simulink model "diosya"  (R2022a)
settings: Solver=FixedStepAuto  StartTime=0.0  StopTime=10.0  RelTol=1e-3
libraries: vexv5lib x61, vexcommonlib x1
settings Model: Creator=alice  LastModifiedBy=alice
settings SolverCC: AlgebraicLoopSolver=TrustRegion
settings DataIOCC: ReturnWorkspaceOutputs=off
settings OptimizationCC: EnhancedBackFolding=on  PassReuseOutputArgsAs=Individual arguments  MaxStackSize=64  OptimizeBlockOrder=speed  DifferentSizesBufferReuse=on  OptimizationCustomize=off  EfficientTunableParamExpr=on
settings DebuggingCC: ParameterTunabilityLossMsg=error  UnconnectedInputMsg=warning  UnconnectedOutputMsg=warning  UnconnectedLineMsg=warning  SFMachineParentedDataDiag=warning  ArithmeticOperatorsInVariantConditions=warning
settings HardwareCC: ProdBitPerPointer=32  ProdBitPerSizeT=32  ProdBitPerPtrDiffT=32  ProdLargestAtomicInteger=Long  ProdLargestAtomicFloat=Double  ProdWordSize=32  ProdHWDeviceType=ARM Compatible->ARM Cortex
settings SFSimCC: MATLABDynamicMemAlloc=off  CustomCodeUndefinedFunction=UseInterfaceOnly
settings RTWCC: SystemTargetFile=ert.tlc  HardwareBoard=VEX V5 Robot Brain  TLCOptions="-aInlineSetEventsForThisBaseRateFcn=TLC_FALSE -aSuppressMultiTaskScheduler=TLC_FALSE  -aRateBasedStepFcn=0"  TemplateMakefile=ert_default_tmf  GenerateReport=on  Toolchain=GNU Tools for ARM Embedded Processors  IncludeHyperlinkInReport=on  LaunchReport=on  GenerateTraceInfo=on  GenerateTraceReport=on  GenerateTraceReportSl=on  GenerateTraceReportSf=on  GenerateTraceReportEml=on
settings CodeAppCC: ForceParamTrailComments=on  IgnoreCustomStorageClasses=off  OperatorAnnotations=on  SimulinkDataObjDesc=on  SFDataObjDesc=on  InsertBlockDesc=on

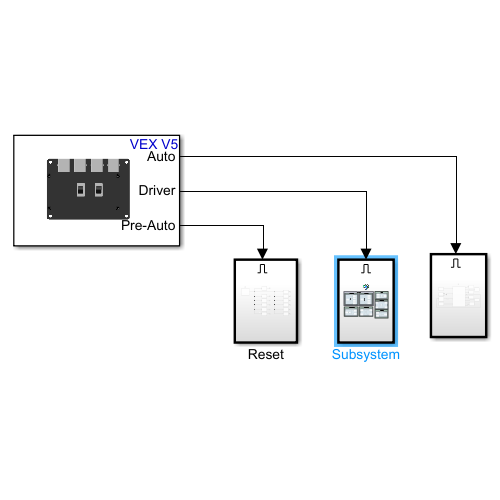
[thumbnail: Simulink's stored preview of the top-level diagram]
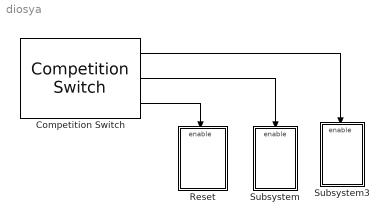
== system diosya ==
  Competition Switch : vexv5lib/Gamepad/Competition Switch  SampleTime=0.02
      settings: SourceProductBaseCode=VEXV5
  Reset : Subsystem
  Subsystem : Subsystem
  Subsystem3 : Subsystem
  wires:
  Competition Switch/1 -> Subsystem3/Enable
  Competition Switch/2 -> Subsystem/Enable
  Competition Switch/3 -> Reset/Enable

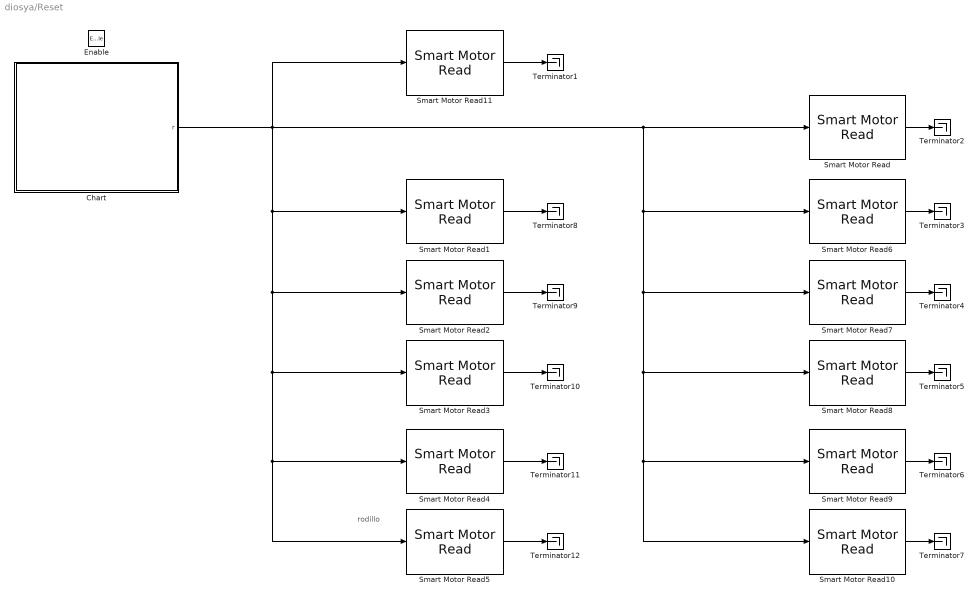
== system diosya/Reset ==
  note: rodillo
  Enable : EnablePort
  Chart : Stateflow chart  TreatAsAtomicUnit=on
  Smart Motor Read : vexv5lib/Sensors/Smart Motor Read  motorPort=2  EncoderUnit=Counts  resetOption=Reset by external signal  additionalOutput=off  SampleTime=0.2
      settings: SourceProductBaseCode=VEXV5
  Smart Motor Read1 : vexv5lib/Sensors/Smart Motor Read  motorPort=10  EncoderUnit=Degrees  resetOption=Reset by external signal  additionalOutput=off  SampleTime=0.2
      settings: SourceProductBaseCode=VEXV5
  Smart Motor Read10 : vexv5lib/Sensors/Smart Motor Read  motorPort=14  EncoderUnit=Degrees  resetOption=Reset by external signal  additionalOutput=off  SampleTime=0.2
      settings: SourceProductBaseCode=VEXV5
  Smart Motor Read11 : vexv5lib/Sensors/Smart Motor Read  motorPort=18  EncoderUnit=Counts  resetOption=Reset by external signal  additionalOutput=off  SampleTime=0.2
      settings: SourceProductBaseCode=VEXV5
  Smart Motor Read2 : vexv5lib/Sensors/Smart Motor Read  motorPort=8  EncoderUnit=Degrees  resetOption=Reset by external signal  additionalOutput=off  SampleTime=0.2
      settings: SourceProductBaseCode=VEXV5
  Smart Motor Read3 : vexv5lib/Sensors/Smart Motor Read  motorPort=9  EncoderUnit=Degrees  resetOption=Reset by external signal  additionalOutput=off  SampleTime=0.2
      settings: SourceProductBaseCode=VEXV5
  Smart Motor Read4 : vexv5lib/Sensors/Smart Motor Read  motorPort=19  EncoderUnit=Degrees  resetOption=Reset by external signal  additionalOutput=off  SampleTime=0.2
      settings: SourceProductBaseCode=VEXV5
  Smart Motor Read5 : vexv5lib/Sensors/Smart Motor Read  motorPort=3  EncoderUnit=Degrees  resetOption=Reset by external signal  additionalOutput=off  SampleTime=0.2
      settings: SourceProductBaseCode=VEXV5
  Smart Motor Read6 : vexv5lib/Sensors/Smart Motor Read  motorPort=7  EncoderUnit=Degrees  resetOption=Reset by external signal  additionalOutput=off  SampleTime=0.2
      settings: SourceProductBaseCode=VEXV5
  Smart Motor Read7 : vexv5lib/Sensors/Smart Motor Read  motorPort=12  EncoderUnit=Degrees  resetOption=Reset by external signal  additionalOutput=off  SampleTime=0.2
      settings: SourceProductBaseCode=VEXV5
  Smart Motor Read8 : vexv5lib/Sensors/Smart Motor Read  motorPort=13  EncoderUnit=Degrees  resetOption=Reset by external signal  additionalOutput=off  SampleTime=0.2
      settings: SourceProductBaseCode=VEXV5
  Smart Motor Read9 : vexv5lib/Sensors/Smart Motor Read  motorPort=17  EncoderUnit=Degrees  resetOption=Reset by external signal  additionalOutput=off  SampleTime=0.2
      settings: SourceProductBaseCode=VEXV5
  Terminator{1..12} (12 alike) : Terminator
  wires:
  Smart Motor Read/1 -> Terminator2/1
  Chart/1(r) -> Smart Motor Read5/1, Smart Motor Read4/1, Smart Motor Read3/1, Smart Motor Read2/1, Smart Motor Read1/1, Smart Motor Read11/1, Smart Motor Read6/1, Smart Motor Read9/1, Smart Motor Read10/1, Smart Motor Read8/1, Smart Motor Read7/1, Smart Motor Read/1
  Smart Motor Read8/1 -> Terminator5/1
  Smart Motor Read4/1 -> Terminator11/1
  Smart Motor Read1/1 -> Terminator8/1
  Smart Motor Read3/1 -> Terminator10/1
  Smart Motor Read9/1 -> Terminator6/1
  Smart Motor Read2/1 -> Terminator9/1
  Smart Motor Read5/1 -> Terminator12/1
  Smart Motor Read10/1 -> Terminator7/1
  Smart Motor Read7/1 -> Terminator4/1
  Smart Motor Read6/1 -> Terminator3/1
  Smart Motor Read11/1 -> Terminator1/1

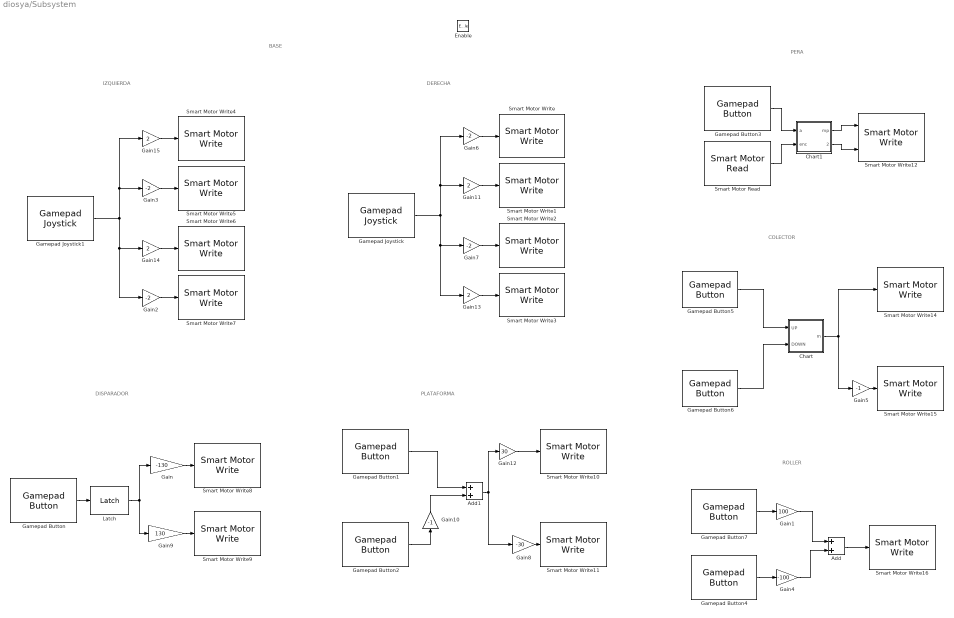
== system diosya/Subsystem ==
  note: PERA
  note: DISPARADOR
  note: DERECHA
  note: ROLLER
  note: BASE
  note: PLATAFORMA
  note: IZQUIERDA
  note: COLECTOR
  Enable : EnablePort
  Add : Sum
  Add1 : Sum
  Chart : Stateflow chart  TreatAsAtomicUnit=on
      settings: PortSchema="{\"entries\":[{\"content\":{\"sides\":[{\"content\":{\"connectorIds\":[\"In2\",\"In1\"]},\"type\":\"ConnectorPlacement.EquallySpacedRectSide\",\"uuid\":\"cbee530c-459d-43ce-b0ca-bbbcd9764774\"},{\"content\":{\"connectorIds\":[\"Out1\"],\"side\":\"RIGHT\"},\"type\":\"ConnectorPlacement.EquallySpacedRectSide\",\"uuid\":\"d644d29c-22a6-445b-a79a-ab4f9a428935\"},{\"content\":{\"connectorIds\":[],\"side\":\"TOP\"},\"type\":\"ConnectorPlacement.EquallySpacedRectSide\",\"uuid\":\"bec18bfc-fa48-4772-9326-1d1444bb53f6\"}]},\"type\":\"ConnectorPlacement.EquallySpacedConnector\",\"uuid\":\"71acd1fe-ef1f-429a-bb10-23fe236c7399\"}],\"packageUris\":[\"http://schema.mathworks.com/mf0/Connector/R2020b\"],\"version\":\"1.0\"}"
  Chart1 : Stateflow chart  TreatAsAtomicUnit=on
  Gain : Gain  Gain=-130
  Gain1 : Gain  Gain=100
  Gain10 : Gain  Gain=-1
  Gain{11,13..15} (4 alike) : Gain  Gain=2
  Gain12 : Gain  Gain=30
  Gain{2..3,6..7} (4 alike) : Gain  Gain=-2
  Gain4 : Gain  Gain=-100
  Gain5 : Gain  Gain=-1
  Gain8 : Gain  Gain=-30
  Gain9 : Gain  Gain=130
  Gamepad Button : vexv5lib/Gamepad/Gamepad Button  joystickType=Primary  chan=A  SampleTime=0.02
      settings: SourceProductBaseCode=VEXV5
  Gamepad Button1 : vexv5lib/Gamepad/Gamepad Button  joystickType=Primary  chan=L1  SampleTime=0.02
      settings: SourceProductBaseCode=VEXV5
  Gamepad Button2 : vexv5lib/Gamepad/Gamepad Button  joystickType=Primary  chan=R1  SampleTime=0.02
      settings: SourceProductBaseCode=VEXV5
  Gamepad Button3 : vexv5lib/Gamepad/Gamepad Button  joystickType=Primary  chan=X  SampleTime=0.02
      settings: SourceProductBaseCode=VEXV5
  Gamepad Button4 : vexv5lib/Gamepad/Gamepad Button  joystickType=Primary  chan=R2  SampleTime=0.02
      settings: SourceProductBaseCode=VEXV5
  Gamepad Button5 : vexv5lib/Gamepad/Gamepad Button  joystickType=Primary  chan=B  SampleTime=0.02
      settings: SourceProductBaseCode=VEXV5
  Gamepad Button6 : vexv5lib/Gamepad/Gamepad Button  joystickType=Primary  chan=DOWN  SampleTime=0.02
      settings: SourceProductBaseCode=VEXV5
  Gamepad Button7 : vexv5lib/Gamepad/Gamepad Button  joystickType=Primary  chan=L2  SampleTime=0.02
      settings: SourceProductBaseCode=VEXV5
  Gamepad Joystick : vexv5lib/Gamepad/Gamepad Joystick  joystickType=Primary  chan=2  SampleTime=0.02
      settings: SourceProductBaseCode=VEXV5
  Gamepad Joystick1 : vexv5lib/Gamepad/Gamepad Joystick  joystickType=Primary  chan=3  SampleTime=0.02
      settings: SourceProductBaseCode=VEXV5
  Latch : vexcommonlib/Latch  output0=off  BlockPlatform=vexv5
      settings: SourceProductBaseCode=EC_VEX_MICRO,VEXV5
  Smart Motor Read : vexv5lib/Sensors/Smart Motor Read  motorPort=18  EncoderUnit=Counts  resetOption=No reset  additionalOutput=off  SampleTime=0.2
      settings: SourceProductBaseCode=VEXV5
  Smart Motor Write : vexv5lib/Actuators/Smart Motor Write  motorPort=2  scaleFactor=18:1  MotorBrakeMode=Coast  OperationMode=Velocity Control
      settings: SourceProductBaseCode=VEXV5
  Smart Motor Write1 : vexv5lib/Actuators/Smart Motor Write  motorPort=7  scaleFactor=18:1  MotorBrakeMode=Coast  OperationMode=Velocity Control
      settings: SourceProductBaseCode=VEXV5
  Smart Motor Write10 : vexv5lib/Actuators/Smart Motor Write  motorPort=17  scaleFactor=36:1  MotorBrakeMode=Hold  OperationMode=Velocity Control
      settings: SourceProductBaseCode=VEXV5
  Smart Motor Write11 : vexv5lib/Actuators/Smart Motor Write  motorPort=14  scaleFactor=36:1  MotorBrakeMode=Hold  OperationMode=Velocity Control
      settings: SourceProductBaseCode=VEXV5
  Smart Motor Write12 : vexv5lib/Actuators/Smart Motor Write  motorPort=18  scaleFactor=18:1  MotorBrakeMode=Coast  OperationMode=Position Control
      settings: SourceProductBaseCode=VEXV5
  Smart Motor Write14 : vexv5lib/Actuators/Smart Motor Write  motorPort=16  scaleFactor=18:1  MotorBrakeMode=Coast  OperationMode=Velocity Control
      settings: SourceProductBaseCode=VEXV5
  Smart Motor Write15 : vexv5lib/Actuators/Smart Motor Write  motorPort=11  scaleFactor=18:1  MotorBrakeMode=Coast  OperationMode=Velocity Control
      settings: SourceProductBaseCode=VEXV5
  Smart Motor Write16 : vexv5lib/Actuators/Smart Motor Write  motorPort=3  scaleFactor=18:1  MotorBrakeMode=Coast  OperationMode=Velocity Control
      settings: SourceProductBaseCode=VEXV5
  Smart Motor Write2 : vexv5lib/Actuators/Smart Motor Write  motorPort=12  scaleFactor=18:1  MotorBrakeMode=Coast  OperationMode=Velocity Control
      settings: SourceProductBaseCode=VEXV5
  Smart Motor Write3 : vexv5lib/Actuators/Smart Motor Write  motorPort=13  scaleFactor=18:1  MotorBrakeMode=Coast  OperationMode=Velocity Control
      settings: SourceProductBaseCode=VEXV5
  Smart Motor Write4 : vexv5lib/Actuators/Smart Motor Write  motorPort=10  scaleFactor=18:1  MotorBrakeMode=Coast  OperationMode=Velocity Control
      settings: SourceProductBaseCode=VEXV5
  Smart Motor Write5 : vexv5lib/Actuators/Smart Motor Write  motorPort=8  scaleFactor=18:1  MotorBrakeMode=Coast  OperationMode=Velocity Control
      settings: SourceProductBaseCode=VEXV5
  Smart Motor Write6 : vexv5lib/Actuators/Smart Motor Write  motorPort=9  scaleFactor=18:1  MotorBrakeMode=Coast  OperationMode=Velocity Control
      settings: SourceProductBaseCode=VEXV5
  Smart Motor Write7 : vexv5lib/Actuators/Smart Motor Write  motorPort=19  scaleFactor=18:1  MotorBrakeMode=Coast  OperationMode=Velocity Control
      settings: SourceProductBaseCode=VEXV5
  Smart Motor Write8 : vexv5lib/Actuators/Smart Motor Write  motorPort=20  scaleFactor=18:1  MotorBrakeMode=Coast  OperationMode=Velocity Control
      settings: SourceProductBaseCode=VEXV5
  Smart Motor Write9 : vexv5lib/Actuators/Smart Motor Write  motorPort=4  scaleFactor=18:1  MotorBrakeMode=Coast  OperationMode=Velocity Control
      settings: SourceProductBaseCode=VEXV5
  wires:
  Gamepad Joystick1/1 -> Gain14/1, Gain2/1, Gain3/1, Gain15/1
  Gain9/1 -> Smart Motor Write9/1
  Gamepad Button4/1 -> Gain4/1
  Add1/1 -> Gain8/1, Gain12/1
  Gamepad Button/1 -> Latch/1
  Gain1/1 -> Add/1
  Gain4/1 -> Add/2
  Chart/1(m) -> Gain5/1, Smart Motor Write14/1
  Add/1 -> Smart Motor Write16/1
  Gamepad Button7/1 -> Gain1/1
  Gain10/1 -> Add1/2
  Gain14/1 -> Smart Motor Write6/1
  Gamepad Button6/1 -> Chart/1(DOWN)
  Gain7/1 -> Smart Motor Write2/1
  Gain11/1 -> Smart Motor Write1/1
  Gain13/1 -> Smart Motor Write3/1
  Gamepad Joystick/1 -> Gain7/1, Gain13/1, Gain11/1, Gain6/1
  Gain8/1 -> Smart Motor Write11/1
  Gamepad Button2/1 -> Gain10/1
  Gain/1 -> Smart Motor Write8/1
  Gain3/1 -> Smart Motor Write5/1
  Gamepad Button3/1 -> Chart1/1(a)
  Gain5/1 -> Smart Motor Write15/1
  Latch/1 -> Gain9/1, Gain/1
  Gamepad Button5/1 -> Chart/2(UP)
  Chart1/1(mp) -> Smart Motor Write12/1
  Chart1/2(position) -> Smart Motor Write12/2
  Smart Motor Read/1 -> Chart1/2(enc)
  Gain15/1 -> Smart Motor Write4/1
  Gain12/1 -> Smart Motor Write10/1
  Gamepad Button1/1 -> Add1/1
  Gain2/1 -> Smart Motor Write7/1
  Gain6/1 -> Smart Motor Write/1

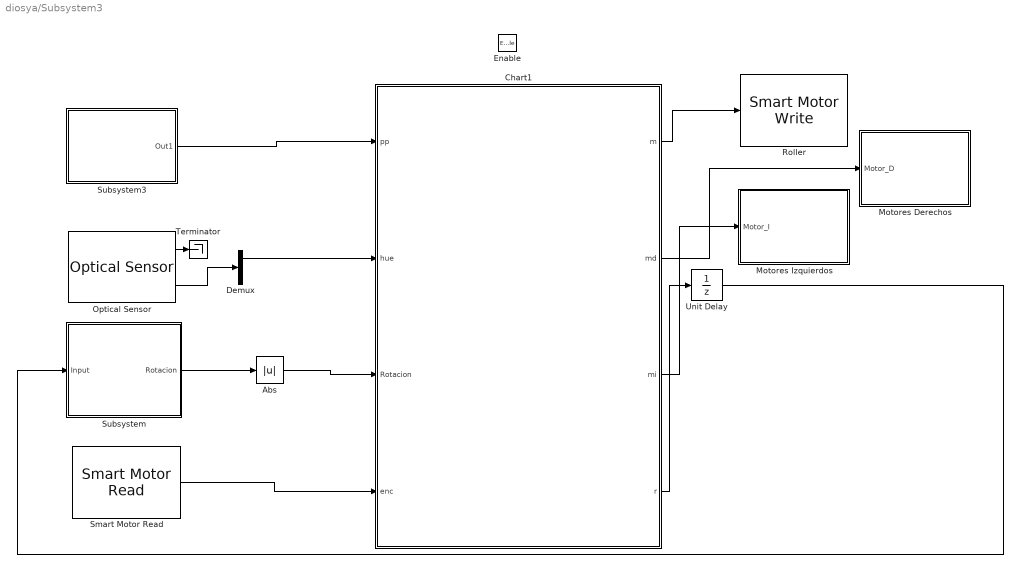
== system diosya/Subsystem3 ==
  Enable : EnablePort
  Abs : Abs  SaturateOnIntegerOverflow=off
  Chart1 : Stateflow chart  TreatAsAtomicUnit=on
      settings: PortSchema="{\"entries\":[{\"content\":{\"sides\":[{\"content\":{\"connectorIds\":[\"In4\",\"In1\",\"In2\",\"In3\"]},\"type\":\"ConnectorPlacement.EquallySpacedRectSide\",\"uuid\":\"6dcbe489-9116-465f-8670-0b6fb9f421dc\"},{\"content\":{\"connectorIds\":[\"Out1\",\"Out2\",\"Out3\",\"Out4\"],\"side\":\"RIGHT\"},\"type\":\"ConnectorPlacement.EquallySpacedRectSide\",\"uuid\":\"705a66a0-558e-4373-baaf-984c25ba8fc1\"},{\"content\":{\"connectorIds\":[],\"side\":\"TOP\"},\"type\":\"ConnectorPlacement.EquallySpacedRectSide\",\"uuid\":\"a9acb6ac-8695-4fbf-8ec3-a93009f982d4\"}]},\"type\":\"ConnectorPlacement.EquallySpacedConnector\",\"uuid\":\"5cef7c66-f869-485c-ad0a-97aa792678b1\"}],\"packageUris\":[\"http://schema.mathworks.com/mf0/Connector/R2020b\"],\"version\":\"1.0\"}"
  Demux : Demux  Outputs=3
  Motores Derechos : Subsystem
  Motores Izquierdos : Subsystem
  Optical Sensor : vexv5lib/Sensors/Optical Sensor  SmartPort=15  Mode=Color  LedPower=100.0  HSBopt=on  RGBopt=off  RawGestureOpt=off  SampleTime=0.1
      settings: SourceProductBaseCode=VEXV5
  Roller : vexv5lib/Actuators/Smart Motor Write  motorPort=3  scaleFactor=18:1  MotorBrakeMode=Brake  OperationMode=Velocity Control
      settings: SourceProductBaseCode=VEXV5
  Smart Motor Read : vexv5lib/Sensors/Smart Motor Read  motorPort=18  EncoderUnit=Counts  resetOption=No reset  additionalOutput=off  SampleTime=0.2
      settings: SourceProductBaseCode=VEXV5
  Subsystem : Subsystem
  Subsystem3 : Subsystem
  Terminator : Terminator
  Unit Delay : UnitDelay  SampleTime=-1  HasFrameUpgradeWarning=on
  wires:
  Chart1/1(m) -> Roller/1
  Optical Sensor/2 -> Demux/1
  Demux/1 -> Chart1/1(hue)
  Optical Sensor/1 -> Terminator/1
  Chart1/2(md) -> Motores Derechos/1(Motor_D)
  Chart1/3(mi) -> Motores Izquierdos/1(Motor_I)
  Subsystem/1(Rotacion) -> Abs/1
  Abs/1 -> Chart1/2(Rotacion)
  Chart1/4(r) -> Unit Delay/1
  Unit Delay/1 -> Subsystem/1(Input)
  Smart Motor Read/1 -> Chart1/3(enc)
  Subsystem3/1(Out1) -> Chart1/4(pp)

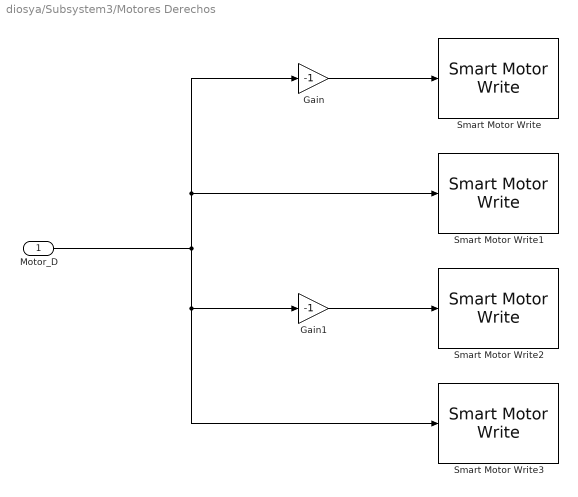
== system diosya/Subsystem3/Motores Derechos ==
  Motor_D : Inport
  Gain : Gain  Gain=-1
  Gain1 : Gain  Gain=-1
  Smart Motor Write : vexv5lib/Actuators/Smart Motor Write  motorPort=2  scaleFactor=36:1  MotorBrakeMode=Brake  OperationMode=Velocity Control
      settings: SourceProductBaseCode=VEXV5
  Smart Motor Write1 : vexv5lib/Actuators/Smart Motor Write  motorPort=7  scaleFactor=36:1  MotorBrakeMode=Brake  OperationMode=Velocity Control
      settings: SourceProductBaseCode=VEXV5
  Smart Motor Write2 : vexv5lib/Actuators/Smart Motor Write  motorPort=12  scaleFactor=36:1  MotorBrakeMode=Brake  OperationMode=Velocity Control
      settings: SourceProductBaseCode=VEXV5
  Smart Motor Write3 : vexv5lib/Actuators/Smart Motor Write  motorPort=13  scaleFactor=36:1  MotorBrakeMode=Brake  OperationMode=Velocity Control
      settings: SourceProductBaseCode=VEXV5
  wires:
  Motor_D/1 -> Smart Motor Write3/1, Gain1/1, Smart Motor Write1/1, Gain/1
  Gain/1 -> Smart Motor Write/1
  Gain1/1 -> Smart Motor Write2/1

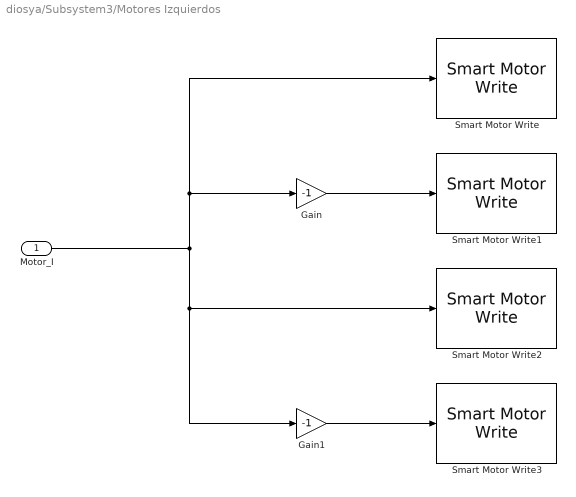
== system diosya/Subsystem3/Motores Izquierdos ==
  Motor_I : Inport
  Gain : Gain  Gain=-1
  Gain1 : Gain  Gain=-1
  Smart Motor Write : vexv5lib/Actuators/Smart Motor Write  motorPort=10  scaleFactor=36:1  MotorBrakeMode=Brake  OperationMode=Velocity Control
      settings: SourceProductBaseCode=VEXV5
  Smart Motor Write1 : vexv5lib/Actuators/Smart Motor Write  motorPort=8  scaleFactor=36:1  MotorBrakeMode=Brake  OperationMode=Velocity Control
      settings: SourceProductBaseCode=VEXV5
  Smart Motor Write2 : vexv5lib/Actuators/Smart Motor Write  motorPort=9  scaleFactor=36:1  MotorBrakeMode=Brake  OperationMode=Velocity Control
      settings: SourceProductBaseCode=VEXV5
  Smart Motor Write3 : vexv5lib/Actuators/Smart Motor Write  motorPort=19  scaleFactor=36:1  MotorBrakeMode=Brake  OperationMode=Velocity Control
      settings: SourceProductBaseCode=VEXV5
  wires:
  Motor_I/1 -> Gain1/1, Smart Motor Write2/1, Gain/1, Smart Motor Write/1
  Gain/1 -> Smart Motor Write1/1
  Gain1/1 -> Smart Motor Write3/1

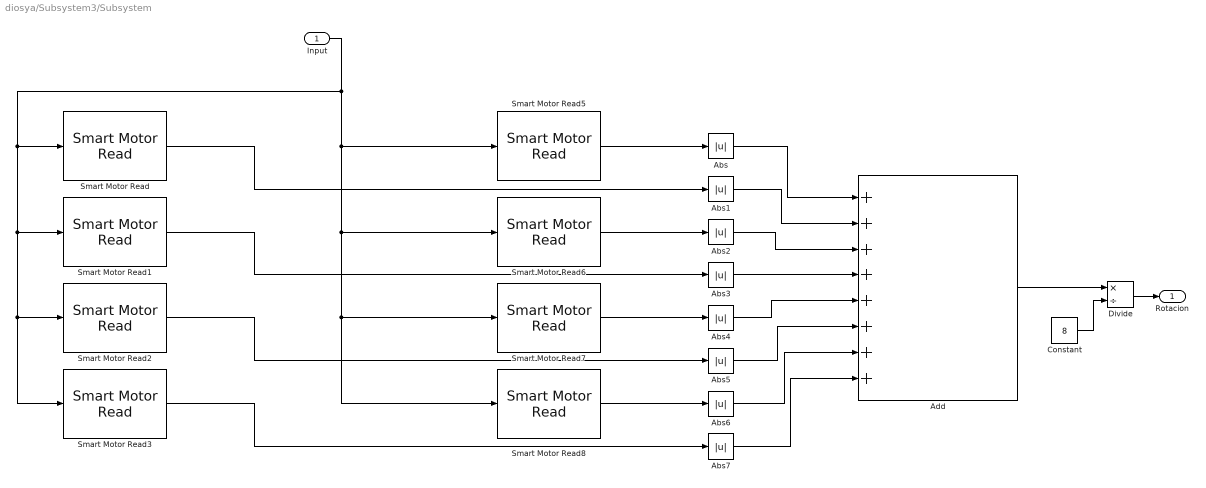
== system diosya/Subsystem3/Subsystem ==
  Input : Inport
  Abs{,1..7} (8 alike) : Abs  SaturateOnIntegerOverflow=off
  Add : Sum  Inputs=++++++++
  Constant : Constant  Value=8
  Divide : Product  Inputs=*/
  Smart Motor Read : vexv5lib/Sensors/Smart Motor Read  motorPort=10  EncoderUnit=Degrees  resetOption=Reset by external signal  additionalOutput=off  SampleTime=0.2
      settings: SourceProductBaseCode=VEXV5
  Smart Motor Read1 : vexv5lib/Sensors/Smart Motor Read  motorPort=8  EncoderUnit=Degrees  resetOption=Reset by external signal  additionalOutput=off  SampleTime=0.2
      settings: SourceProductBaseCode=VEXV5
  Smart Motor Read2 : vexv5lib/Sensors/Smart Motor Read  motorPort=9  EncoderUnit=Degrees  resetOption=Reset by external signal  additionalOutput=off  SampleTime=0.2
      settings: SourceProductBaseCode=VEXV5
  Smart Motor Read3 : vexv5lib/Sensors/Smart Motor Read  motorPort=19  EncoderUnit=Degrees  resetOption=Reset by external signal  additionalOutput=off  SampleTime=0.2
      settings: SourceProductBaseCode=VEXV5
  Smart Motor Read5 : vexv5lib/Sensors/Smart Motor Read  motorPort=2  EncoderUnit=Degrees  resetOption=Reset by external signal  additionalOutput=off  SampleTime=0.2
      settings: SourceProductBaseCode=VEXV5
  Smart Motor Read6 : vexv5lib/Sensors/Smart Motor Read  motorPort=7  EncoderUnit=Degrees  resetOption=Reset by external signal  additionalOutput=off  SampleTime=0.2
      settings: SourceProductBaseCode=VEXV5
  Smart Motor Read7 : vexv5lib/Sensors/Smart Motor Read  motorPort=12  EncoderUnit=Degrees  resetOption=Reset by external signal  additionalOutput=off  SampleTime=0.2
      settings: SourceProductBaseCode=VEXV5
  Smart Motor Read8 : vexv5lib/Sensors/Smart Motor Read  motorPort=13  EncoderUnit=Degrees  resetOption=Reset by external signal  additionalOutput=off  SampleTime=0.2
      settings: SourceProductBaseCode=VEXV5
  Rotacion : Outport
  wires:
  Input/1 -> Smart Motor Read8/1, Smart Motor Read7/1, Smart Motor Read6/1, Smart Motor Read5/1, Smart Motor Read/1, Smart Motor Read3/1, Smart Motor Read2/1, Smart Motor Read1/1
  Smart Motor Read5/1 -> Abs/1
  Add/1 -> Divide/1
  Constant/1 -> Divide/2
  Divide/1 -> Rotacion/1
  Abs/1 -> Add/1
  Abs1/1 -> Add/2
  Abs2/1 -> Add/3
  Abs3/1 -> Add/4
  Abs4/1 -> Add/5
  Abs5/1 -> Add/6
  Abs6/1 -> Add/7
  Abs7/1 -> Add/8
  Smart Motor Read/1 -> Abs1/1
  Smart Motor Read6/1 -> Abs2/1
  Smart Motor Read1/1 -> Abs3/1
  Smart Motor Read7/1 -> Abs4/1
  Smart Motor Read2/1 -> Abs5/1
  Smart Motor Read8/1 -> Abs6/1
  Smart Motor Read3/1 -> Abs7/1

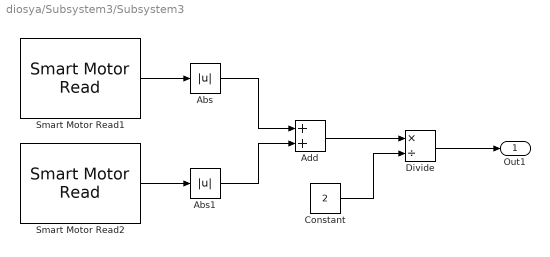
== system diosya/Subsystem3/Subsystem3 ==
  Abs : Abs  SaturateOnIntegerOverflow=off
  Abs1 : Abs  SaturateOnIntegerOverflow=off
  Add : Sum
  Constant : Constant  Value=2
  Divide : Product  Inputs=*/
  Smart Motor Read1 : vexv5lib/Sensors/Smart Motor Read  motorPort=17  EncoderUnit=Counts  resetOption=No reset  additionalOutput=off  SampleTime=0.2
      settings: SourceProductBaseCode=VEXV5
  Smart Motor Read2 : vexv5lib/Sensors/Smart Motor Read  motorPort=14  EncoderUnit=Counts  resetOption=No reset  additionalOutput=off  SampleTime=0.2
      settings: SourceProductBaseCode=VEXV5
  Out1 : Outport
  wires:
  Smart Motor Read1/1 -> Abs/1
  Smart Motor Read2/1 -> Abs1/1
  Abs/1 -> Add/1
  Abs1/1 -> Add/2
  Add/1 -> Divide/1
  Constant/1 -> Divide/2
  Divide/1 -> Out1/1

== stateflow chart diosya/Subsystem/Chart ==
  state SOLTAR
    during:
    m=-200;
  state INICIO
    entry:
    m=0;
  state AGARRAR
    during:
    m=200;
  state YESYES
    during:
    m=-200;
  state YES
    during:
    m=-200;
  state KEEP
    during:
    m=200;
  state KEEPKEEP
    during:
    m=200;
  KEEPKEEP -> INICIO : after(0.2,sec)
  YESYES -> INICIO : after(0.2,sec)
  (default) -> INICIO
  INICIO -> SOLTAR [order 2] : [DOWN == 1]
  INICIO -> AGARRAR [order 1] : [UP == 1]
  SOLTAR -> YES : [DOWN == 0]
  AGARRAR -> KEEP : [UP == 0]
  YES -> KEEP [order 1] : [UP == 1]
  YES -> YESYES [order 2] : [DOWN == 1]
  KEEP -> KEEPKEEP [order 2] : [UP == 1]
  KEEP -> YES [order 1] : [DOWN == 1]
  data: m output; DOWN input; UP input

== stateflow chart diosya/Subsystem/Chart1 ==
  state LANZAR
    during:
    position=-500;
    enc==position;
    mp=-200;
  state REGRESAR
    during:
    position=0;
    enc==position;
    mp=180;
  state INICIO
    entry:
    position=0;
    mp=0;
  (default) -> INICIO
  LANZAR -> REGRESAR : after(0.5,sec)
  INICIO -> LANZAR : [a==1]
  REGRESAR -> INICIO : after(0.5,sec)
  data: a input; enc input; mp output; position output

== stateflow chart diosya/Subsystem3/Chart1 ==
  state MOVERAZUL
    during:
    m = -10;
    mi=-2; md=-2;
  state YEET
    during:
    m=0; mi=0;
    md=0; r=1;
  state INICIO
    entry:
    mi=0; md=0;
    r=1;
  state STOP2
    during:
    r=0; mi=0;
    md=0;
  state PAROFINAL
    during:
    r=0; mi=0;
    md=0;
  state VUELTA
    during:
    mi=20;
    md=-20; r=0;
  state PAROO
    during:
    mi=0; md=0;
    r=1;
  state AVANCE
    during:
    mi=20;
    md=20; r=0;
  state MOVERROJO
    during:
    m = -20;
    mi=-2; md=-2;
  state STOP
    during:
    m=0; mi=0;
    md=0; r=1;
  state CANASTA
    during:
    mi=0;
    md=0;
  state VUELTA2
    during:
    mi=-30;
    md=30; r=0;
  state PARITO
    during:
    mi=0;
    md=0; r=1;
  STOP2 -> MOVERAZUL [order 1] : [hue > 210 && hue < 260]
  MOVERAZUL -> YEET : [(hue > 250 && hue < 350)||after(2,sec)]
  YEET -> PAROFINAL : after(0.5,sec)
  (default) -> INICIO
  PAROO -> AVANCE : after(0.5,sec)
  VUELTA -> PAROO : [Rotacion >= 100]
  INICIO -> STOP2 : after(0.5,sec)
  PAROFINAL -> VUELTA : after(0.5,sec)
  STOP2 -> MOVERROJO [order 2] : [hue < 30]
  STOP -> PAROFINAL : after(0.5,sec)
  AVANCE -> PARITO : [Rotacion >= 350]
  MOVERROJO -> STOP : [(hue > 220 && hue < 358)||after(2,sec)]
  VUELTA2 -> CANASTA : [Rotacion >= 100]
  PARITO -> VUELTA2 : after(0.5,sec)
  data: hue input; m output; md output; mi output; r output; Rotacion input; enc input; pp input

== stateflow chart diosya/Reset/Chart ==
  state INICIO
    during:
    r=1;
  state STOP
    during:
    r=0;
  (default) -> INICIO
  INICIO -> STOP : after(1,sec)
  data: r output
